simulink model "aquapack_9_5"  (R2026a)
settings: Solver=FixedStepDiscrete  StopTime=10000
undefined symbols (not defined in the file or in its folder): j
libraries: hdlsllib x22, simulink x5
settings Model: DataTypeOverride=Off  Creator=Aweso  LastModifiedBy=Aweso
settings DataIOCC: InspectSignalLogs=on
settings OptimizationCC: ConditionallyExecuteInputs=off
settings DebuggingCC: SignalRangeChecking=warning  AlgebraicLoopMsg=error  SingleTaskRateTransMsg=error  ParameterPrecisionLossMsg=none  StrictBusMsg=ErrorOnBusTreatedAsVector
settings HardwareCC: ProdHWDeviceType=ASIC/FPGA->ASIC/FPGA  TargetBitPerLong=64.0  TargetBitPerPointer=64.0  TargetBitPerSizeT=64.0  TargetBitPerPtrDiffT=64.0  TargetIntDivRoundTo=Zero  TargetEndianess=LittleEndian  TargetWordSize=64.0  TargetHWDeviceType=AMD->Athlon 64  ProdEqTarget=off
settings ConfigComp: CovScope=ReferencedModels

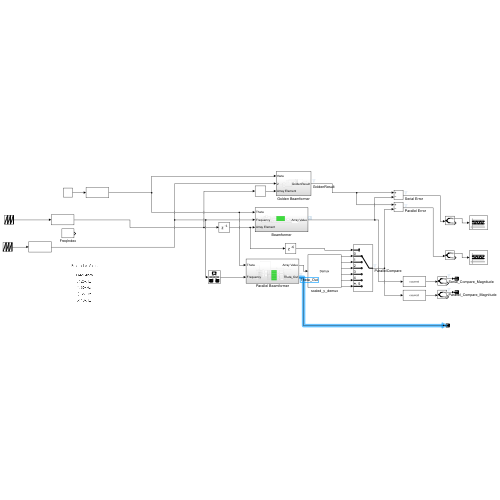
[thumbnail: Simulink's stored preview of the top-level diagram]
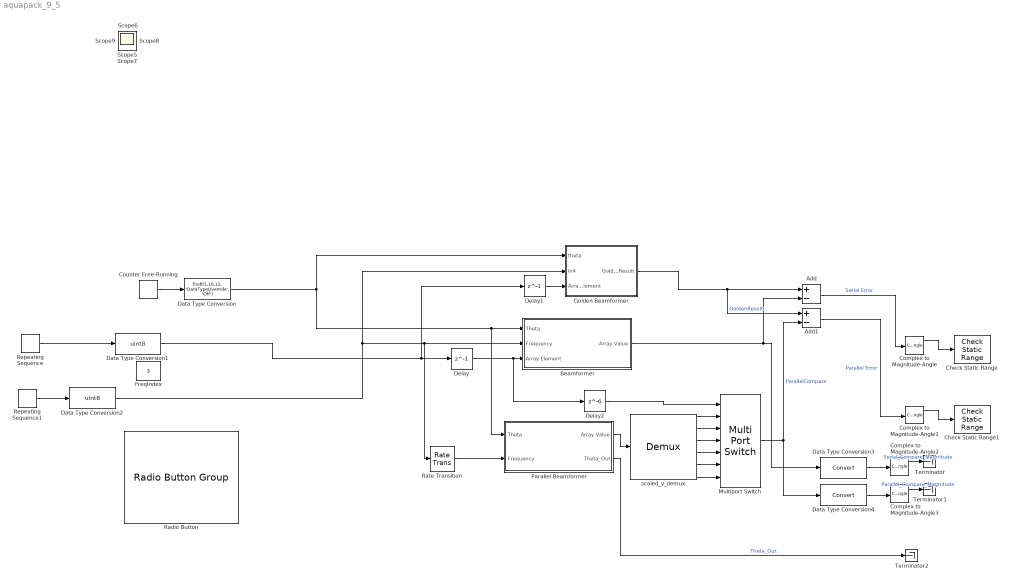
== system aquapack_9_5 ==
  Add : Sum  Inputs=+-
  Add1 : Sum  Inputs=+-
  Beamformer : Subsystem
  Check Static Range : simulink/Model Verification/Check  Static Range  Description=-1 <= u <= 1  max=1  max_included=on  min=-1  min_included=on  enabled=on  stopWhenAssertionFail=on  export=off  icon=graphic
  Check Static Range1 : simulink/Model Verification/Check  Static Range  Description=-1 <= u <= 1  max=1  max_included=on  min=-1  min_included=on  enabled=on  stopWhenAssertionFail=on  export=off  icon=graphic
  Complex to Magnitude-Angle{,1..3} (4 alike) : ComplexToMagnitudeAngle
  Counter Free-Running : simulink/Sources/Counter Free-Running  NumBits=16  tsamp=1000/4096
  Data Type Conversion : DataTypeConversion  OutMin=[-2*pi]  OutMax=[2*pi]  OutDataTypeStr=fixdt(1,16,12, 'DataTypeOverride', 'Off')  ConvertRealWorld=Stored Integer (SI)  SaturateOnIntegerOverflow=off  RndMeth=Floor
  Data Type Conversion1 : DataTypeConversion  OutDataTypeStr=uint8  ConvertRealWorld=Stored Integer (SI)  SaturateOnIntegerOverflow=off  RndMeth=Floor
  Data Type Conversion2 : DataTypeConversion  OutDataTypeStr=uint8  ConvertRealWorld=Stored Integer (SI)  SaturateOnIntegerOverflow=off  RndMeth=Floor
  Data Type Conversion3 : DataTypeConversion  SaturateOnIntegerOverflow=off  RndMeth=Floor
  Data Type Conversion4 : DataTypeConversion  SaturateOnIntegerOverflow=off  RndMeth=Floor
  Delay : Delay  DelayLength=1  InitialCondition=0
  Delay1 : Delay  DelayLength=1  InitialCondition=0
  Delay2 : Delay  DelayLength=6  InitialCondition=0
  FreqIndex : Constant  Value=3  OutDataTypeStr=Inherit: Inherit via back propagation  SampleTime=-1
  Golden Beamformer : Subsystem
  Multiport Switch : MultiPortSwitch  DataPortOrder=Zero-based contiguous  Inputs=6  zeroidx=on  OutDataTypeStr=Inherit: Inherit via back propagation  SaturateOnIntegerOverflow=off  InputSameDT=off
  Parallel Beamformer : Subsystem
  Radio Button : RadioButtonGroup  SelectedLabel=40kHz  ButtonGroupName=Frequency
  Rate Transition : RateTransition  OutPortSampleTimeOpt=Inherit
  Repeating Sequence : simulink/Sources/Repeating Sequence  rep_seq_t=[0 1000 2000 3000 4000 5000 6000]  rep_seq_y=[0 1 2 3 4 5 6]
  Repeating Sequence1 : simulink/Sources/Repeating Sequence  rep_seq_t=[0 6000 12000 18000 24000]  rep_seq_y=[0 1 2 3 4]
  Terminator : Terminator
  Terminator1 : Terminator
  Terminator2 : Terminator
  scaled_y_demux : Demux  Outputs=6
      settings: DisplayOption=none
  Scope{,1..9} (10 alike) : Scope
      Scope settings: ActiveDisplayYMinimum=-2.570616323502799  ActiveDisplayYMaximum=9.0026644172130439
      Scope2 settings: ActiveDisplayYMinimum=-9.37737375181548E+246  ActiveDisplayYMaximum=8.4396363766339327E+247  DataLoggingVariableName=ScopeData2
      Scope3 settings: ActiveDisplayYMinimum=-3207.7499999999991  ActiveDisplayYMaximum=28869.75  DataLoggingVariableName=ScopeData3
      Scope4 settings: ActiveDisplayYMinimum=-1.2498855590820312  ActiveDisplayYMaximum=1.2495803833007812  DataLoggingVariableName=ScopeData5
      Scope5 settings: ActiveDisplayYMinimum=-0.044877976179122925  ActiveDisplayYMaximum=0.044877976179122925  DataLoggingVariableName=ScopeData6
      Scope6 settings: ActiveDisplayYMinimum=-0.0016140900546877468  ActiveDisplayYMaximum=0.00037267566531830429  DataLoggingVariableName=ScopeData7
      Scope7 settings: ActiveDisplayYMinimum=-5.0456498388829193E-14  ActiveDisplayYMaximum=4.954350161117081E-14  DataLoggingVariableName=ScopeData8
      Scope8 settings: ActiveDisplayYMinimum=-6.2795698768761712  ActiveDisplayYMaximum=5.99869519393901  DataLoggingVariableName=ScopeData9
      Scope9 settings: DataLoggingVariableName=ScopeData10
  wires:
  Counter Free-Running/1 -> Data Type Conversion/1
  Golden Beamformer/1(GoldenResult) -> Add1/1, Add/1  "GoldenResult"
  Beamformer/1(Array Value) -> Data Type Conversion3/1, Add/2
  Data Type Conversion/1 -> Golden Beamformer/1(theta), Parallel Beamformer/1(Theta), Beamformer/1(Theta)
  Delay/1 -> Delay2/1, Beamformer/3(Array Element)
  Data Type Conversion1/1 -> Delay1/1, Delay/1
  Repeating Sequence/1 -> Data Type Conversion1/1
  Delay1/1 -> Golden Beamformer/3(Array Element)
  Repeating Sequence1/1 -> Data Type Conversion2/1
  Parallel Beamformer/1(Array Value) -> scaled_y_demux/1
  scaled_y_demux/1 -> Multiport Switch/2
  scaled_y_demux/2 -> Multiport Switch/3
  scaled_y_demux/3 -> Multiport Switch/4
  scaled_y_demux/4 -> Multiport Switch/5
  scaled_y_demux/5 -> Multiport Switch/6
  scaled_y_demux/6 -> Multiport Switch/7
  Delay2/1 -> Multiport Switch/1
  Multiport Switch/1 -> Add1/2, Data Type Conversion4/1  "ParallelCompare"
  Add1/1 -> Complex to Magnitude-Angle1/1  "Parallel Error"
  Add/1 -> Complex to Magnitude-Angle/1  "Serial Error"
  Complex to Magnitude-Angle/1 -> Check Static Range/1
  Complex to Magnitude-Angle1/1 -> Check Static Range1/1
  Complex to Magnitude-Angle2/1 -> Terminator/1  "Serial_Compare_Magnitude"
  Complex to Magnitude-Angle3/1 -> Terminator1/1  "Parallel_Compare_Magnitude"
  Data Type Conversion3/1 -> Complex to Magnitude-Angle2/1
  Data Type Conversion4/1 -> Complex to Magnitude-Angle3/1
  Rate Transition/1 -> Parallel Beamformer/2(Frequency)
  Data Type Conversion2/1 -> Golden Beamformer/2(In4), Beamformer/2(Frequency), Rate Transition/1
  Parallel Beamformer/2(Theta_Out) -> Terminator2/1  "Theta_Out"

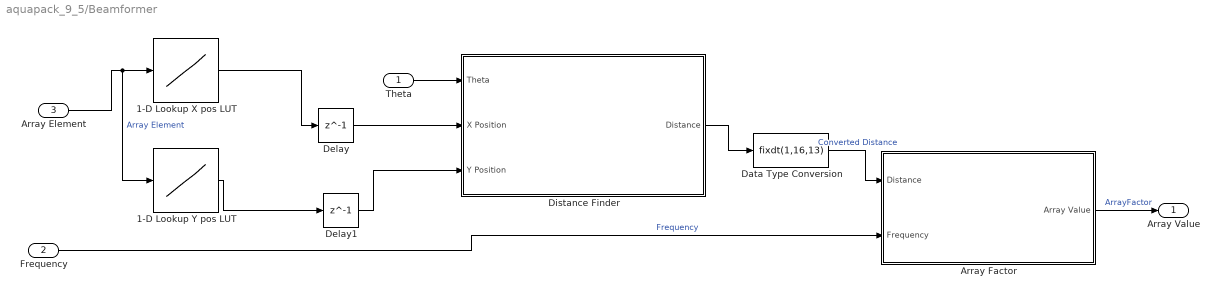
== system aquapack_9_5/Beamformer ==
  Theta : Inport
  Frequency : Inport  Port=2
  Array Element : Inport  Port=3
  1-D Lookup X pos LUT : Lookup_n-D  NumberOfTableDimensions=1  BreakpointsForDimension1=[0 1 2 3 4 5]  BreakpointsForDimension1DataTypeStr=uint8  IndexSearchMethod=Linear search  Table=|  InterpMethod=Flat  InternalRulePriority=Speed  OutDataTypeStr=Inherit: Inherit via back propagation  RndMeth=Simplest
      | [0.025400000000000
      | 0.007849031657124
      | -0.020549031657124
      | -0.020549031657124
      | 0.007849031657124
      | 0]
  1-D Lookup Y pos LUT : Lookup_n-D  NumberOfTableDimensions=1  BreakpointsForDimension1=[0 1 2 3 4 5]  BreakpointsForDimension1DataTypeStr=uint8  IndexSearchMethod=Linear search  Table=|  InterpMethod=Flat  InternalRulePriority=Speed  OutDataTypeStr=Inherit: Inherit via back propagation  RndMeth=Simplest
      | [0
      | 0.024156835513897
      | 0.014929745408229
      | -0.014929745408229
      | -0.024156835513897
      | 0]
  Array Factor : Subsystem
  Data Type Conversion : DataTypeConversion  OutMin=[-2]  OutMax=[2]  OutDataTypeStr=fixdt(1,16,13)  SaturateOnIntegerOverflow=off  RndMeth=Floor
  Delay : Delay  DelayLength=1  InitialCondition=0
  Delay1 : Delay  DelayLength=1  InitialCondition=0
  Distance Finder : Subsystem
  Array Value : Outport
  wires:
  1-D Lookup X pos LUT/1 -> Delay/1
  Frequency/1 -> Array Factor/2(Frequency)  "Frequency"
  1-D Lookup Y pos LUT/1 -> Delay1/1
  Theta/1 -> Distance Finder/1(Theta)
  Array Factor/1(Array Value) -> Array Value/1  "ArrayFactor"
  Distance Finder/1(Distance) -> Data Type Conversion/1
  Data Type Conversion/1 -> Array Factor/1(Distance)  "Converted Distance"
  Array Element/1 -> 1-D Lookup Y pos LUT/1, 1-D Lookup X pos LUT/1  "Array Element"
  Delay/1 -> Distance Finder/2(X Position)
  Delay1/1 -> Distance Finder/3(Y Position)

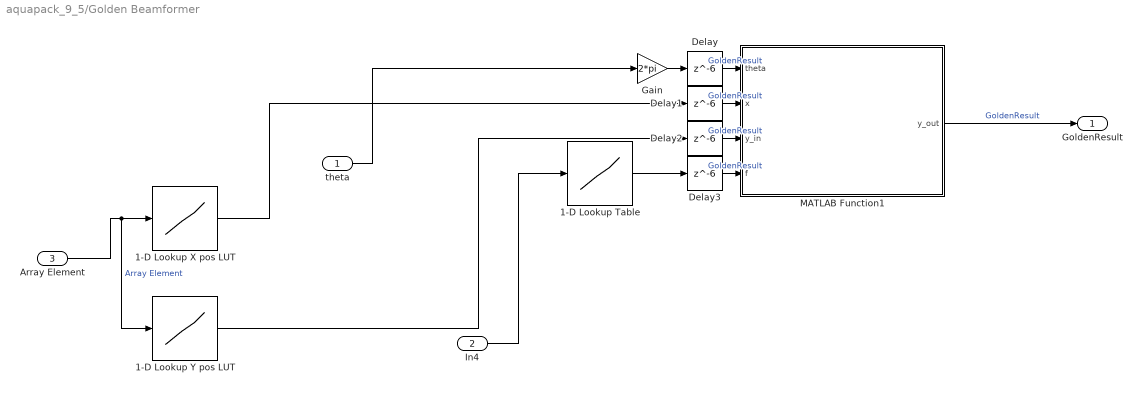
== system aquapack_9_5/Golden Beamformer ==
  theta : Inport
  In4 : Inport  Port=2
  Array Element : Inport  Port=3
  1-D Lookup Table : Lookup_n-D  NumberOfTableDimensions=1  LookupTableObject=''  BreakpointsForDimension1=0:3  BreakpointsForDimension1FirstPoint=10  BreakpointsForDimension2FirstPoint=10  BreakpointsForDimension1Spacing=12  BreakpointsForDimension2Spacing=12  BreakpointsForDimension1DataTypeStr=uint8  IndexSearchMethod=Evenly spaced points  Table=(25e3:5e3:40e3) * 2*pi/1480  InterpMethod=Flat  DiagnosticForOutOfRangeInput=Error  InternalRulePriority=Speed  OutMin=[106.13]  OutMax=[,169.82]  OutDataTypeStr=fixdt(1,16,7)  RndMeth=Simplest
  1-D Lookup X pos LUT : Lookup_n-D  NumberOfTableDimensions=1  BreakpointsForDimension1=[0 1 2 3 4 5]  IndexSearchMethod=Linear search  Table=|  InterpMethod=Flat  InternalRulePriority=Speed  OutDataTypeStr=double  RndMeth=Simplest
      | [0.025400000000000
      | 0.007849031657124
      | -0.020549031657124
      | -0.020549031657124
      | 0.007849031657124
      | 0]
  1-D Lookup Y pos LUT : Lookup_n-D  NumberOfTableDimensions=1  BreakpointsForDimension1=[0 1 2 3 4 5]  IndexSearchMethod=Linear search  Table=|  InterpMethod=Flat  InternalRulePriority=Speed  OutDataTypeStr=double  RndMeth=Simplest
      | [0
      | 0.024156835513897
      | 0.014929745408229
      | -0.014929745408229
      | -0.024156835513897
      | 0]
  Delay{,1..3} (4 alike) : Delay  DelayLength=6  InitialCondition=0
  Gain : Gain  Gain=2*pi
  MATLAB Function1 : MATLAB Function  TreatAsAtomicUnit=on
  GoldenResult : Outport
  wires:
  1-D Lookup X pos LUT/1 -> Delay1/1
  1-D Lookup Table/1 -> Delay3/1
  In4/1 -> 1-D Lookup Table/1
  theta/1 -> Gain/1
  1-D Lookup Y pos LUT/1 -> Delay2/1
  MATLAB Function1/1(y_out) -> GoldenResult/1  "GoldenResult"
  Delay/1 -> MATLAB Function1/1(theta)  "GoldenResult"
  Delay1/1 -> MATLAB Function1/2(x)  "GoldenResult"
  Delay2/1 -> MATLAB Function1/3(y_in)  "GoldenResult"
  Delay3/1 -> MATLAB Function1/4(f)  "GoldenResult"
  Gain/1 -> Delay/1
  Array Element/1 -> 1-D Lookup Y pos LUT/1, 1-D Lookup X pos LUT/1  "Array Element"

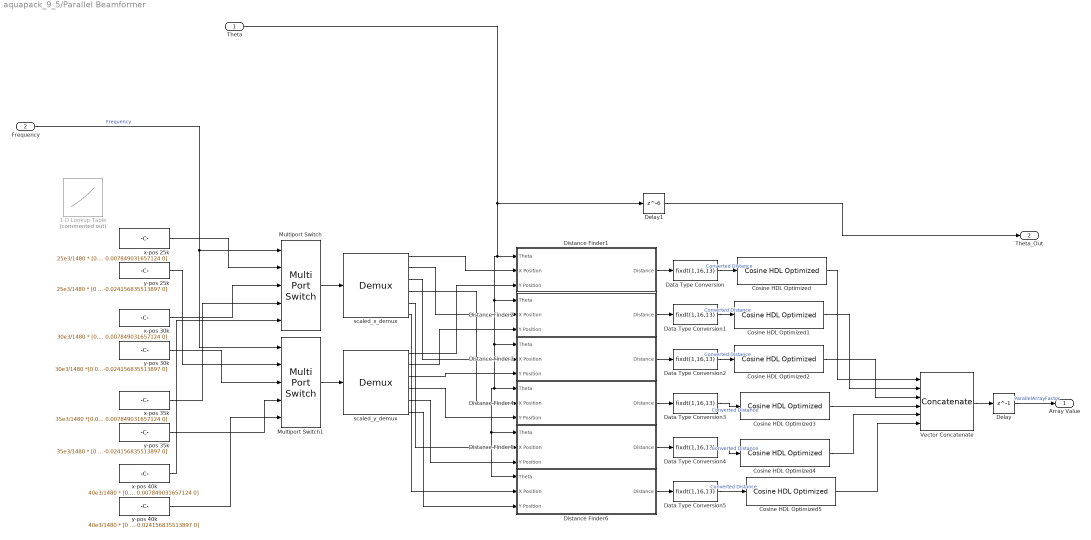
== system aquapack_9_5/Parallel Beamformer ==
  Theta : Inport
  Frequency : Inport  Port=2
  1-D Lookup Table : Lookup_n-D  Commented=on  NumberOfTableDimensions=1  LookupTableObject=''  BreakpointsForDimension1=0:3  BreakpointsForDimension1FirstPoint=10  BreakpointsForDimension2FirstPoint=10  BreakpointsForDimension1Spacing=12  BreakpointsForDimension2Spacing=12  BreakpointsForDimension1DataTypeStr=uint8  IndexSearchMethod=Evenly spaced points  Table=(25e3:5e3:40e3)/1480  InterpMethod=Flat  DiagnosticForOutOfRangeInput=Error  InternalRulePriority=Speed  OutMin=[106.13]  OutMax=[,169.82]  OutDataTypeStr=fixdt(1,16,7)  RndMeth=Simplest  InputSameDT=off
  Cosine HDL Optimized{,1..5} (6 alike) : hdlsllib/Lookup Tables/Cosine HDL Optimized  OutputFormula=exp(j*2*pi*u)  NumDataPoints=512  TableDataTypeStr=fixdt(1,16,15)  SimulateLUTROMDelay=on
  Data Type Conversion{,1..5} (6 alike) : DataTypeConversion  OutMin=[-2]  OutMax=[2]  OutDataTypeStr=fixdt(1,16,13)  SaturateOnIntegerOverflow=off  RndMeth=Floor
  Delay : Delay  DelayLength=1
  Delay1 : Delay  DelayLength=6
  Distance Finder1 : Subsystem
  Distance Finder2 : Subsystem
  Distance Finder3 : Subsystem
  Distance Finder4 : Subsystem
  Distance Finder5 : Subsystem
  Distance Finder6 : Subsystem
  Multiport Switch : MultiPortSwitch  DataPortOrder=Zero-based contiguous  Inputs=4  zeroidx=on  OutDataTypeStr=Inherit: Inherit via back propagation  SaturateOnIntegerOverflow=off  InputSameDT=off
  Multiport Switch1 : MultiPortSwitch  DataPortOrder=Zero-based contiguous  Inputs=4  zeroidx=on  OutDataTypeStr=Inherit: Inherit via back propagation  SaturateOnIntegerOverflow=off  InputSameDT=off
  Vector Concatenate : Concatenate  NumInputs=6
  scaled_x_demux : Demux  Outputs=6
      settings: DisplayOption=none
  scaled_y_demux : Demux  Outputs=6
      settings: DisplayOption=none
  x-pos 25k : Constant  Value=|  OutDataTypeStr=Inherit: Inherit via back propagation
      | 25e3/1480 * [0.025400000000000
      | 0.007849031657124
      | -0.020549031657124
      | -0.020549031657124
      | 0.007849031657124
      | 0]
  x-pos 30k : Constant  Value=|  OutDataTypeStr=Inherit: Inherit via back propagation
      | 30e3/1480 * [0.025400000000000
      | 0.007849031657124
      | -0.020549031657124
      | -0.020549031657124
      | 0.007849031657124
      | 0]
  x-pos 35k : Constant  Value=|  OutDataTypeStr=Inherit: Inherit via back propagation
      | 35e3/1480 *[0.025400000000000
      | 0.007849031657124
      | -0.020549031657124
      | -0.020549031657124
      | 0.007849031657124
      | 0]
  x-pos 40k : Constant  Value=|  OutDataTypeStr=Inherit: Inherit via back propagation
      | 40e3/1480 * [0.025400000000000
      | 0.007849031657124
      | -0.020549031657124
      | -0.020549031657124
      | 0.007849031657124
      | 0]
  y-pos 25k : Constant  Value=|  OutDataTypeStr=Inherit: Inherit via back propagation
      | 25e3/1480 * [0
      | 0.024156835513897
      | 0.014929745408229
      | -0.014929745408229
      | -0.024156835513897
      | 0]
  y-pos 30k : Constant  Value=|  OutDataTypeStr=Inherit: Inherit via back propagation
      | 30e3/1480 *[0
      | 0.024156835513897
      | 0.014929745408229
      | -0.014929745408229
      | -0.024156835513897
      | 0]
  y-pos 35k : Constant  Value=|  OutDataTypeStr=Inherit: Inherit via back propagation
      | 35e3/1480 * [0
      | 0.024156835513897
      | 0.014929745408229
      | -0.014929745408229
      | -0.024156835513897
      | 0]
  y-pos 40k : Constant  Value=|  OutDataTypeStr=Inherit: Inherit via back propagation
      | 40e3/1480 * [0
      | 0.024156835513897
      | 0.014929745408229
      | -0.014929745408229
      | -0.024156835513897
      | 0]
  Array Value : Outport
  Theta_Out : Outport  Port=2
  wires:
  Delay/1 -> Array Value/1  "ParallelArrayFactor"
  x-pos 25k/1 -> Multiport Switch/2
  x-pos 30k/1 -> Multiport Switch/3
  x-pos 35k/1 -> Multiport Switch/4
  x-pos 40k/1 -> Multiport Switch/5
  y-pos 25k/1 -> Multiport Switch1/2
  y-pos 30k/1 -> Multiport Switch1/3
  y-pos 35k/1 -> Multiport Switch1/4
  y-pos 40k/1 -> Multiport Switch1/5
  Multiport Switch/1 -> scaled_x_demux/1
  Multiport Switch1/1 -> scaled_y_demux/1
  Frequency/1 -> Multiport Switch1/1, Multiport Switch/1  "Frequency"
  scaled_x_demux/2 -> Distance Finder2/2(X Position)
  scaled_x_demux/3 -> Distance Finder3/2(X Position)
  scaled_x_demux/4 -> Distance Finder4/2(X Position)
  scaled_x_demux/5 -> Distance Finder5/2(X Position)
  scaled_x_demux/6 -> Distance Finder6/2(X Position)
  scaled_y_demux/1 -> Distance Finder1/3(Y Position)
  scaled_y_demux/2 -> Distance Finder2/3(Y Position)
  scaled_y_demux/3 -> Distance Finder3/3(Y Position)
  scaled_y_demux/4 -> Distance Finder4/3(Y Position)
  scaled_y_demux/5 -> Distance Finder5/3(Y Position)
  scaled_y_demux/6 -> Distance Finder6/3(Y Position)
  Theta/1 -> Delay1/1, Distance Finder2/1(Theta), Distance Finder3/1(Theta), Distance Finder4/1(Theta), Distance Finder6/1(Theta), Distance Finder5/1(Theta), Distance Finder1/1(Theta)
  Distance Finder2/1(Distance) -> Data Type Conversion1/1
  Distance Finder1/1(Distance) -> Data Type Conversion/1
  Distance Finder3/1(Distance) -> Data Type Conversion2/1
  Distance Finder4/1(Distance) -> Data Type Conversion3/1
  Distance Finder5/1(Distance) -> Data Type Conversion4/1
  Distance Finder6/1(Distance) -> Data Type Conversion5/1
  Data Type Conversion5/1 -> Cosine HDL Optimized5/1  "Converted Distance"
  Data Type Conversion/1 -> Cosine HDL Optimized/1  "Converted Distance"
  Data Type Conversion1/1 -> Cosine HDL Optimized1/1  "Converted Distance"
  Data Type Conversion2/1 -> Cosine HDL Optimized2/1  "Converted Distance"
  Data Type Conversion3/1 -> Cosine HDL Optimized3/1  "Converted Distance"
  Data Type Conversion4/1 -> Cosine HDL Optimized4/1  "Converted Distance"
  Cosine HDL Optimized5/1 -> Vector Concatenate/6
  Cosine HDL Optimized4/1 -> Vector Concatenate/5
  Cosine HDL Optimized3/1 -> Vector Concatenate/4
  Cosine HDL Optimized2/1 -> Vector Concatenate/3
  Cosine HDL Optimized1/1 -> Vector Concatenate/2
  Cosine HDL Optimized/1 -> Vector Concatenate/1
  Vector Concatenate/1 -> Delay/1
  scaled_x_demux/1 -> Distance Finder1/2(X Position)
  Delay1/1 -> Theta_Out/1

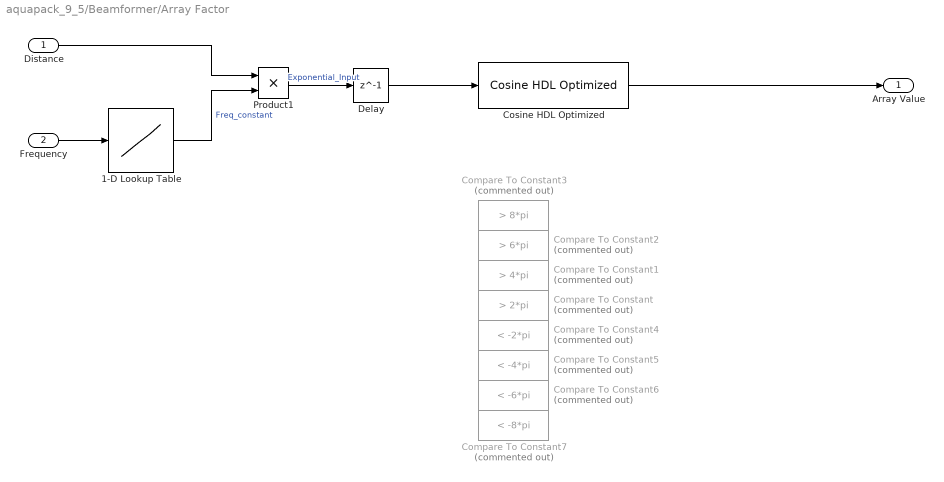
== system aquapack_9_5/Beamformer/Array Factor ==
  Distance : Inport
  Frequency : Inport  Port=2
  1-D Lookup Table : Lookup_n-D  NumberOfTableDimensions=1  LookupTableObject=''  BreakpointsForDimension1=0:3  BreakpointsForDimension1FirstPoint=10  BreakpointsForDimension2FirstPoint=10  BreakpointsForDimension1Spacing=12  BreakpointsForDimension2Spacing=12  BreakpointsForDimension1DataTypeStr=uint8  IndexSearchMethod=Evenly spaced points  Table=(25e3:5e3:40e3)/1480  InterpMethod=Flat  DiagnosticForOutOfRangeInput=Error  InternalRulePriority=Speed  OutMin=[106.13]  OutMax=[,169.82]  OutDataTypeStr=fixdt(1,16,7)  RndMeth=Simplest  InputSameDT=off
  Compare To Constant : hdlsllib/Logic and Bit Operations/Compare To Constant  Commented=on  relop=>  const=2*pi  OutDataTypeStr=boolean
  Compare To Constant1 : hdlsllib/Logic and Bit Operations/Compare To Constant  Commented=on  relop=>  const=4*pi  OutDataTypeStr=boolean
  Compare To Constant2 : hdlsllib/Logic and Bit Operations/Compare To Constant  Commented=on  relop=>  const=6*pi  OutDataTypeStr=boolean
  Compare To Constant3 : hdlsllib/Logic and Bit Operations/Compare To Constant  Commented=on  relop=>  const=8*pi  OutDataTypeStr=boolean
  Compare To Constant4 : hdlsllib/Logic and Bit Operations/Compare To Constant  Commented=on  relop=<  const=-2*pi  OutDataTypeStr=boolean
  Compare To Constant5 : hdlsllib/Logic and Bit Operations/Compare To Constant  Commented=on  relop=<  const=-4*pi  OutDataTypeStr=boolean
  Compare To Constant6 : hdlsllib/Logic and Bit Operations/Compare To Constant  Commented=on  relop=<  const=-6*pi  OutDataTypeStr=boolean
  Compare To Constant7 : hdlsllib/Logic and Bit Operations/Compare To Constant  Commented=on  relop=<  const=-8*pi  OutDataTypeStr=boolean
  Cosine HDL Optimized : hdlsllib/Lookup Tables/Cosine HDL Optimized  OutputFormula=exp(j*2*pi*u)  NumDataPoints=512  TableDataTypeStr=fixdt(1,16,15)  SimulateLUTROMDelay=on
  Delay : Delay  DelayLength=1
  Product1 : Product  OutMin=[-170]  OutMax=[170]  OutDataTypeStr=fixdt(1,16,7)
  Array Value : Outport
  wires:
  Cosine HDL Optimized/1 -> Array Value/1
  Distance/1 -> Product1/1
  Product1/1 -> Delay/1  "Exponential_Input"
  Frequency/1 -> 1-D Lookup Table/1
  1-D Lookup Table/1 -> Product1/2  "Freq_constant"
  Delay/1 -> Cosine HDL Optimized/1

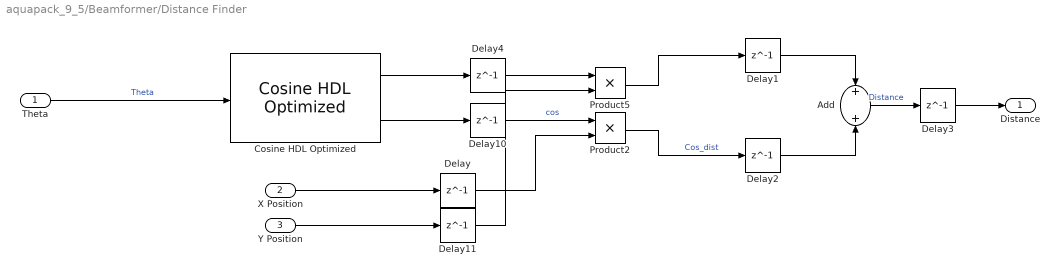
== system aquapack_9_5/Beamformer/Distance Finder ==
  Theta : Inport
  X Position : Inport  Port=2
  Y Position : Inport  Port=3
  Add : Sum
  Cosine HDL Optimized : hdlsllib/Lookup Tables/Cosine HDL Optimized  OutputFormula=sin(2*pi*u) and cos(2*pi*u)  NumDataPoints=512  TableDataTypeStr=fixdt(0,16,15)  SimulateLUTROMDelay=on
  Delay{,1..4,10..11} (7 alike) : Delay  DelayLength=1
  Product2 : Product  InputSameDT=on  OutDataTypeStr=Inherit: Same as first input
  Product5 : Product  InputSameDT=on  OutDataTypeStr=Inherit: Same as first input
  Distance : Outport
  wires:
  X Position/1 -> Delay/1
  Y Position/1 -> Delay11/1
  Add/1 -> Delay3/1  "Distance"
  Product5/1 -> Delay1/1
  Product2/1 -> Delay2/1  "Cos_dist"
  Delay1/1 -> Add/1
  Delay2/1 -> Add/2
  Delay3/1 -> Distance/1
  Theta/1 -> Cosine HDL Optimized/1  "Theta"
  Cosine HDL Optimized/2 -> Delay10/1
  Cosine HDL Optimized/1 -> Delay4/1
  Delay4/1 -> Product5/1
  Delay10/1 -> Product2/1  "cos"
  Delay/1 -> Product2/2
  Delay11/1 -> Product5/2

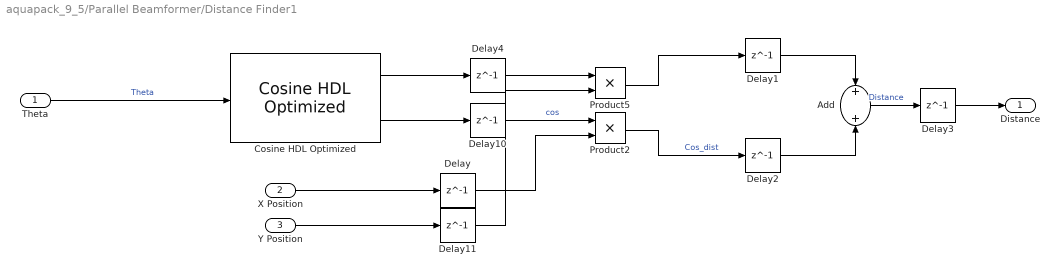
== system aquapack_9_5/Parallel Beamformer/Distance Finder1 ==
  Theta : Inport
  X Position : Inport  Port=2
  Y Position : Inport  Port=3
  Add : Sum
  Cosine HDL Optimized : hdlsllib/Lookup Tables/Cosine HDL Optimized  OutputFormula=sin(2*pi*u) and cos(2*pi*u)  NumDataPoints=512  TableDataTypeStr=fixdt(0,16,15)  SimulateLUTROMDelay=on
  Delay{,1..4,10..11} (7 alike) : Delay  DelayLength=1
  Product2 : Product  InputSameDT=on  OutDataTypeStr=Inherit: Same as first input
  Product5 : Product  InputSameDT=on  OutDataTypeStr=Inherit: Same as first input
  Distance : Outport
  wires:
  X Position/1 -> Delay/1
  Y Position/1 -> Delay11/1
  Add/1 -> Delay3/1  "Distance"
  Product5/1 -> Delay1/1
  Product2/1 -> Delay2/1  "Cos_dist"
  Delay1/1 -> Add/1
  Delay2/1 -> Add/2
  Delay3/1 -> Distance/1
  Theta/1 -> Cosine HDL Optimized/1  "Theta"
  Cosine HDL Optimized/2 -> Delay10/1
  Cosine HDL Optimized/1 -> Delay4/1
  Delay4/1 -> Product5/1
  Delay10/1 -> Product2/1  "cos"
  Delay/1 -> Product2/2
  Delay11/1 -> Product5/2

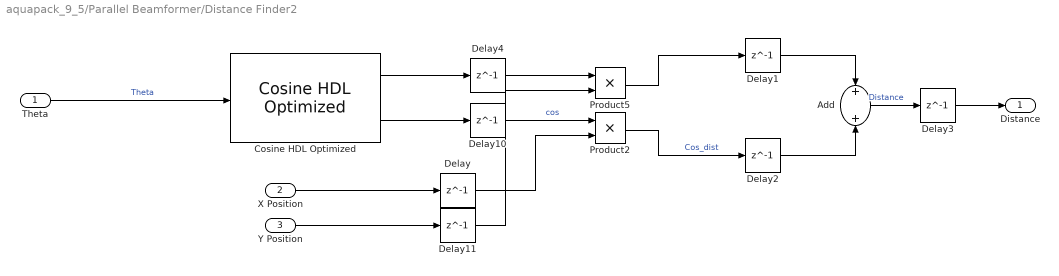
== system aquapack_9_5/Parallel Beamformer/Distance Finder2 ==
  Theta : Inport
  X Position : Inport  Port=2
  Y Position : Inport  Port=3
  Add : Sum
  Cosine HDL Optimized : hdlsllib/Lookup Tables/Cosine HDL Optimized  OutputFormula=sin(2*pi*u) and cos(2*pi*u)  NumDataPoints=512  TableDataTypeStr=fixdt(0,16,15)  SimulateLUTROMDelay=on
  Delay{,1..4,10..11} (7 alike) : Delay  DelayLength=1
  Product2 : Product  InputSameDT=on  OutDataTypeStr=Inherit: Same as first input
  Product5 : Product  InputSameDT=on  OutDataTypeStr=Inherit: Same as first input
  Distance : Outport
  wires:
  X Position/1 -> Delay/1
  Y Position/1 -> Delay11/1
  Add/1 -> Delay3/1  "Distance"
  Product5/1 -> Delay1/1
  Product2/1 -> Delay2/1  "Cos_dist"
  Delay1/1 -> Add/1
  Delay2/1 -> Add/2
  Delay3/1 -> Distance/1
  Theta/1 -> Cosine HDL Optimized/1  "Theta"
  Cosine HDL Optimized/2 -> Delay10/1
  Cosine HDL Optimized/1 -> Delay4/1
  Delay4/1 -> Product5/1
  Delay10/1 -> Product2/1  "cos"
  Delay/1 -> Product2/2
  Delay11/1 -> Product5/2

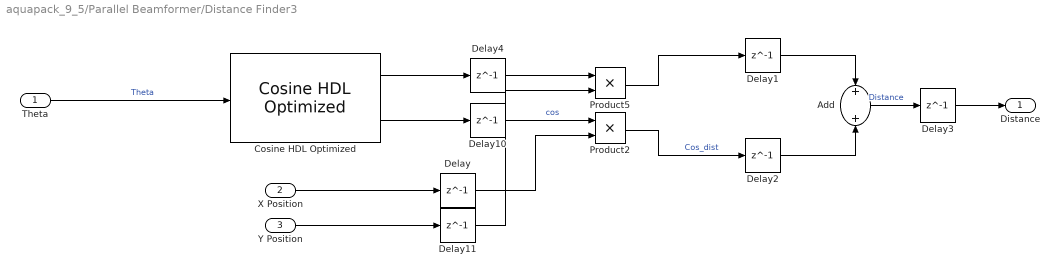
== system aquapack_9_5/Parallel Beamformer/Distance Finder3 ==
  Theta : Inport
  X Position : Inport  Port=2
  Y Position : Inport  Port=3
  Add : Sum
  Cosine HDL Optimized : hdlsllib/Lookup Tables/Cosine HDL Optimized  OutputFormula=sin(2*pi*u) and cos(2*pi*u)  NumDataPoints=512  TableDataTypeStr=fixdt(0,16,15)  SimulateLUTROMDelay=on
  Delay{,1..4,10..11} (7 alike) : Delay  DelayLength=1
  Product2 : Product  InputSameDT=on  OutDataTypeStr=Inherit: Same as first input
  Product5 : Product  InputSameDT=on  OutDataTypeStr=Inherit: Same as first input
  Distance : Outport
  wires:
  X Position/1 -> Delay/1
  Y Position/1 -> Delay11/1
  Add/1 -> Delay3/1  "Distance"
  Product5/1 -> Delay1/1
  Product2/1 -> Delay2/1  "Cos_dist"
  Delay1/1 -> Add/1
  Delay2/1 -> Add/2
  Delay3/1 -> Distance/1
  Theta/1 -> Cosine HDL Optimized/1  "Theta"
  Cosine HDL Optimized/2 -> Delay10/1
  Cosine HDL Optimized/1 -> Delay4/1
  Delay4/1 -> Product5/1
  Delay10/1 -> Product2/1  "cos"
  Delay/1 -> Product2/2
  Delay11/1 -> Product5/2

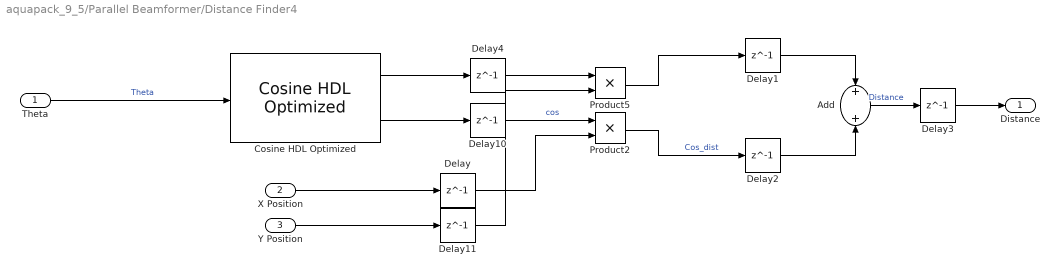
== system aquapack_9_5/Parallel Beamformer/Distance Finder4 ==
  Theta : Inport
  X Position : Inport  Port=2
  Y Position : Inport  Port=3
  Add : Sum
  Cosine HDL Optimized : hdlsllib/Lookup Tables/Cosine HDL Optimized  OutputFormula=sin(2*pi*u) and cos(2*pi*u)  NumDataPoints=512  TableDataTypeStr=fixdt(0,16,15)  SimulateLUTROMDelay=on
  Delay{,1..4,10..11} (7 alike) : Delay  DelayLength=1
  Product2 : Product  InputSameDT=on  OutDataTypeStr=Inherit: Same as first input
  Product5 : Product  InputSameDT=on  OutDataTypeStr=Inherit: Same as first input
  Distance : Outport
  wires:
  X Position/1 -> Delay/1
  Y Position/1 -> Delay11/1
  Add/1 -> Delay3/1  "Distance"
  Product5/1 -> Delay1/1
  Product2/1 -> Delay2/1  "Cos_dist"
  Delay1/1 -> Add/1
  Delay2/1 -> Add/2
  Delay3/1 -> Distance/1
  Theta/1 -> Cosine HDL Optimized/1  "Theta"
  Cosine HDL Optimized/2 -> Delay10/1
  Cosine HDL Optimized/1 -> Delay4/1
  Delay4/1 -> Product5/1
  Delay10/1 -> Product2/1  "cos"
  Delay/1 -> Product2/2
  Delay11/1 -> Product5/2

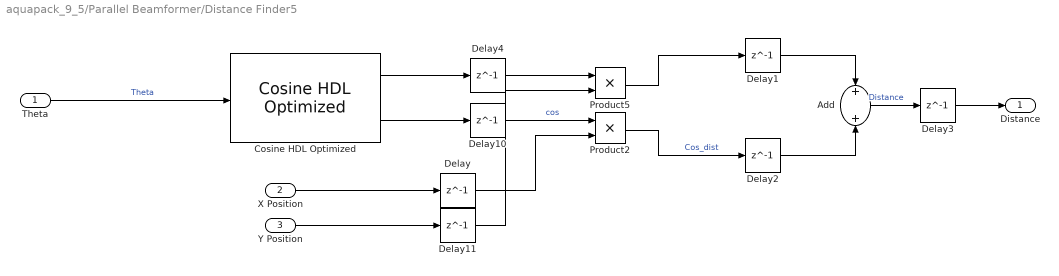
== system aquapack_9_5/Parallel Beamformer/Distance Finder5 ==
  Theta : Inport
  X Position : Inport  Port=2
  Y Position : Inport  Port=3
  Add : Sum
  Cosine HDL Optimized : hdlsllib/Lookup Tables/Cosine HDL Optimized  OutputFormula=sin(2*pi*u) and cos(2*pi*u)  NumDataPoints=512  TableDataTypeStr=fixdt(0,16,15)  SimulateLUTROMDelay=on
  Delay{,1..4,10..11} (7 alike) : Delay  DelayLength=1
  Product2 : Product  InputSameDT=on  OutDataTypeStr=Inherit: Same as first input
  Product5 : Product  InputSameDT=on  OutDataTypeStr=Inherit: Same as first input
  Distance : Outport
  wires:
  X Position/1 -> Delay/1
  Y Position/1 -> Delay11/1
  Add/1 -> Delay3/1  "Distance"
  Product5/1 -> Delay1/1
  Product2/1 -> Delay2/1  "Cos_dist"
  Delay1/1 -> Add/1
  Delay2/1 -> Add/2
  Delay3/1 -> Distance/1
  Theta/1 -> Cosine HDL Optimized/1  "Theta"
  Cosine HDL Optimized/2 -> Delay10/1
  Cosine HDL Optimized/1 -> Delay4/1
  Delay4/1 -> Product5/1
  Delay10/1 -> Product2/1  "cos"
  Delay/1 -> Product2/2
  Delay11/1 -> Product5/2

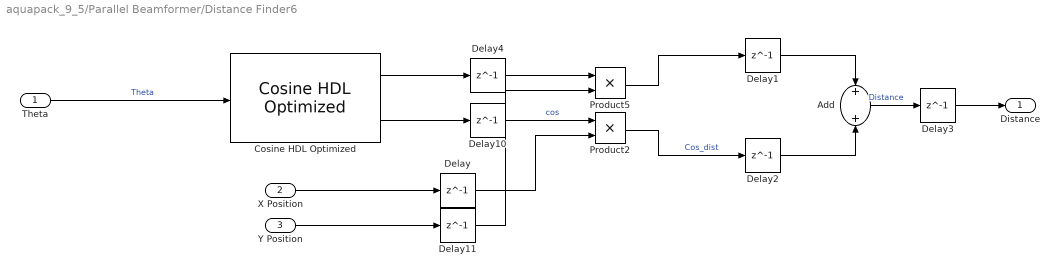
== system aquapack_9_5/Parallel Beamformer/Distance Finder6 ==
  Theta : Inport
  X Position : Inport  Port=2
  Y Position : Inport  Port=3
  Add : Sum
  Cosine HDL Optimized : hdlsllib/Lookup Tables/Cosine HDL Optimized  OutputFormula=sin(2*pi*u) and cos(2*pi*u)  NumDataPoints=512  TableDataTypeStr=fixdt(0,16,15)  SimulateLUTROMDelay=on
  Delay{,1..4,10..11} (7 alike) : Delay  DelayLength=1
  Product2 : Product  InputSameDT=on  OutDataTypeStr=Inherit: Same as first input
  Product5 : Product  InputSameDT=on  OutDataTypeStr=Inherit: Same as first input
  Distance : Outport
  wires:
  X Position/1 -> Delay/1
  Y Position/1 -> Delay11/1
  Add/1 -> Delay3/1  "Distance"
  Product5/1 -> Delay1/1
  Product2/1 -> Delay2/1  "Cos_dist"
  Delay1/1 -> Add/1
  Delay2/1 -> Add/2
  Delay3/1 -> Distance/1
  Theta/1 -> Cosine HDL Optimized/1  "Theta"
  Cosine HDL Optimized/2 -> Delay10/1
  Cosine HDL Optimized/1 -> Delay4/1
  Delay4/1 -> Product5/1
  Delay10/1 -> Product2/1  "cos"
  Delay/1 -> Product2/2
  Delay11/1 -> Product5/2

== matlab function aquapack_9_5/Golden Beamformer/MATLAB Function1 ==
  data: theta input; y_out output; x input; y_in input; f input
function y_out = fcn(theta,x,y_in,f)
% Cast to double for math functions
theta = double(theta);
x     = double(x);
y_in  = double(y_in);
f     = double(f);

dist = sin(theta).*y_in + cos(theta).*x;
y_out = exp(1j * dist .* f);
end
